simulink model "Battery_model_2D_Battery1"  (R2026a)
settings: Solver=VariableStepAuto  StopTime=10000
InitFcn:
  | %% Universal Parameters
  | 
  | Cycle_num = 1000; % number of cycles
  | 
  | Temp_state = 35;
  | 
  | 
  | SoC_state = 0.5;
  | 
  | OCV = [ 3.0025,3.4635,3.521,3.5618,3.6058,3.6426,3.6725,3.7049,3.7486,3.79951,3.8418,3.8738 ,3.9044,3.9448,3.9813,4.0222 ,4.0498,4.0658,4.0919,4.1359,4.2];
  | 
  | 
  | % Cn = 540; % As
  | Ru = 3.19; % KW^-1
  | Rc = 1.94; % KW^-1
  | Cc = 62.7; % JK^-1
  | Cs = 4.5;  % JK^-1
  | 
  | Ea = 31500;  % J * mol^-1
  | eta = 152.5; % unitless
  | Ic = 9000;   % [1/s] normalized current rate
  | Rg = 8.314;  % J / K / mol
  | z = 0.57;    % Ah power law exponent
  | 
  | 
  | 
  | %% Breakpoints
  | Temp = [5, 15, 25, 35, 45];
  | SoC  = [0, 0.05, 0.10, 0.15, 0.20, 0.25, 0.30, 0.35, 0.40, 0.45, 0.50, 0.55, 0.60, 0.65, 0.70, 0.75, 0.80, 0.85, 0.90, 0.95, 1.00];
  | 
  | %% ── CHARGING Parameters ──────────────────────────────────────────────────────
  | 
  | % --- R0 (charge) ---
  | R0_5_ch  = [0.09098063, 0.09098063, 0.09098063, 0.07729039, 0.07041201, 0.07506999, 0.09974696 ...
  |              0.10355653, 0.10333513, 0.10371531, 0.10352259, 0.10328822, 0.10331602, 0.10342002 ...
  |              0.10364672, 0.10394453, 0.10423533, 0.10413898, 0.10372082, 0.10352712, 0.10300533];
  | R0_15_ch  = [0.12804680, 0.12804680, 0.12804680, 0.10877905, 0.09909838, 0.10565405, 0.14038460 ...
  |              0.14574622, 0.14543462, 0.14596969, 0.14569844, 0.14536859, 0.14540772, 0.14555409 ...
  |              0.14587315, 0.14629229, 0.14670156, 0.14656596, 0.14597744, 0.14570482, 0.14497046];
  | R0_25_ch  = [0.15714834, 0.15714834, 0.15714834, 0.13350157, 0.12162074, 0.12966634, 0.17229020 ...
  |              0.17887036, 0.17848795, 0.17914462, 0.17881173, 0.17840691, 0.17845493, 0.17863457 ...
  |              0.17902614, 0.17954054, 0.18004283, 0.17987641, 0.17915414, 0.17881956, 0.17791829];
  | R0_35_ch  = [0.19207020, 0.19207020, 0.19207020, 0.16316858, 0.14864757, 0.15848107, 0.21057691 ...
  |              0.21861932, 0.21815193, 0.21895454, 0.21854766, 0.21805289, 0.21811158, 0.21833114 ...
  |              0.21880973, 0.21943844, 0.22005234, 0.21984894, 0.21896616, 0.21855723, 0.21745569];
  | R0_45_ch  = [0.21607897, 0.21607897, 0.21607897, 0.18356466, 0.16722852, 0.17829121, 0.23689902 ...
  |              0.24594674, 0.24542093, 0.24632386, 0.24586613, 0.24530950, 0.24537554, 0.24562254 ...
  |              0.24616095, 0.24686825, 0.24755889, 0.24733007, 0.24633694, 0.24587689, 0.24463765];
  | R0_ch = [R0_5_ch; R0_15_ch; R0_25_ch; R0_35_ch; R0_45_ch];
  | 
  | % --- R1 (charge) ---
  | R1_5_ch  = [0.02042370, 0.02042370, 0.02077370, 0.01704263, 0.01499740, 0.01607981, 0.02204645 ...
  |              0.02311272, 0.02295408, 0.02251460, 0.02241361, 0.02224373, 0.02204869, 0.02198763 ...
  |              0.02193720, 0.02188186, 0.02186556, 0.02196136, 0.02204788, 0.02216615, 0.02233881];
  | R1_15_ch  = [0.03713400, 0.03713400, 0.03777036, 0.03098661, 0.02726801, 0.02923601, 0.04008445 ...
  |              0.04202312, 0.04173470, 0.04093563, 0.04075202, 0.04044315, 0.04008853, 0.03997751 ...
  |              0.03988582, 0.03978519, 0.03975555, 0.03992974, 0.04008704, 0.04030208, 0.04061602];
  | R1_25_ch  = [0.05835343, 0.05835343, 0.05935343, 0.04869324, 0.04284973, 0.04594231, 0.06298985 ...
  |              0.06603633, 0.06558310, 0.06432742, 0.06403890, 0.06355352, 0.06299626, 0.06282180 ...
  |              0.06267773, 0.06251959, 0.06247302, 0.06274674, 0.06299393, 0.06333184, 0.06382517];
  | R1_35_ch  = [0.08169480, 0.08169480, 0.08309480, 0.06817054, 0.05998962, 0.06431924, 0.08818579 ...
  |              0.09245087, 0.09181634, 0.09005839, 0.08965446, 0.08897493, 0.08819477, 0.08795052 ...
  |              0.08774882, 0.08752743, 0.08746222, 0.08784544, 0.08819150, 0.08866458, 0.08935524];
  | R1_45_ch  = [0.09283500, 0.09283500, 0.09442590, 0.07746652, 0.06817002, 0.07309004, 0.10021113 ...
  |              0.10505781, 0.10433675, 0.10233908, 0.10188006, 0.10110787, 0.10022133, 0.09994378 ...
  |              0.09971457, 0.09946299, 0.09938889, 0.09982437, 0.10021762, 0.10075521, 0.10154005];
  | R1_ch = [R1_5_ch; R1_15_ch; R1_25_ch; R1_35_ch; R1_45_ch];
  | 
  | % --- C1 (charge) ---
  | C1_5_ch  = [0.00131968, 0.00131968, 0.00371968, 0.00485103, 0.00496080, 0.00442106, 0.00227620 ...
  |              0.00183668, 0.00180689, 0.00187453, 0.00180955, 0.00174851, 0.00174631, 0.00176395 ...
  |              0.00179412, 0.00181842, 0.00185225, 0.00188926, 0.00185128, 0.00180647, 0.00169075];
  | C1_15_ch  = [0.00079181, 0.00079181, 0.00223181, 0.00291062, 0.00297648, 0.00265264, 0.00136572 ...
  |              0.00110201, 0.00108413, 0.00112472, 0.00108573, 0.00104911, 0.00104778, 0.00105837 ...
  |              0.00107647, 0.00109105, 0.00111135, 0.00113356, 0.00111077, 0.00108388, 0.00101445];
  | C1_25_ch  = [0.00054987, 0.00054987, 0.00154987, 0.00202126, 0.00206700, 0.00184211, 0.00094842 ...
  |              0.00076528, 0.00075287, 0.00078105, 0.00075398, 0.00072855, 0.00072763, 0.00073498 ...
  |              0.00074755, 0.00075768, 0.00077177, 0.00078719, 0.00077137, 0.00075270, 0.00070448];
  | C1_35_ch  = [0.00040398, 0.00040398, 0.00113868, 0.00148501, 0.00151861, 0.00135339, 0.00069680 ...
  |              0.00056225, 0.00055313, 0.00057383, 0.00055394, 0.00053526, 0.00053458, 0.00053998 ...
  |              0.00054922, 0.00055666, 0.00056701, 0.00057834, 0.00056672, 0.00055300, 0.00051758];
  | C1_45_ch  = [0.00035348, 0.00035348, 0.00099634, 0.00129938, 0.00132879, 0.00118421, 0.00060970 ...
  |              0.00049197, 0.00048399, 0.00050210, 0.00048470, 0.00046835, 0.00046776, 0.00047249 ...
  |              0.00048057, 0.00048708, 0.00049614, 0.00050605, 0.00049588, 0.00048388, 0.00045288];
  | C1_ch = [C1_5_ch; C1_15_ch; C1_25_ch; C1_35_ch; C1_45_ch];
  | 
  | % --- R2 (charge) ---
  | R2_5_ch  = [0.11513467, 0.11513467, 0.11572467, 0.08930958, 0.07499462, 0.08137577, 0.11786696 ...
  |              0.12356614, 0.12135259, 0.11255792, 0.11155202, 0.10963847, 0.10666546, 0.10530908 ...
  |              0.10344252, 0.10111039, 0.09966464, 0.09882254, 0.09857888, 0.09907923, 0.10050567];
  | R2_15_ch  = [0.15351291, 0.15351291, 0.15429957, 0.11907944, 0.09999283, 0.10850103, 0.15715596 ...
  |              0.16475486, 0.16180346, 0.15007724, 0.14873603, 0.14618463, 0.14222061, 0.14041211 ...
  |              0.13792336, 0.13481386, 0.13288620, 0.13176339, 0.13143851, 0.13210565, 0.13400756];
  | R2_25_ch  = [0.19514352, 0.19514352, 0.19614352, 0.15137217, 0.12710953, 0.13792503, 0.19977451 ...
  |              0.20943414, 0.20568235, 0.19077614, 0.18907121, 0.18582791, 0.18078891, 0.17848997 ...
  |              0.17532630, 0.17137355, 0.16892312, 0.16749583, 0.16708284, 0.16793090, 0.17034859];
  | R2_35_ch  = [0.23026935, 0.23026935, 0.23144935, 0.17861916, 0.14998924, 0.16275153, 0.23573393 ...
  |              0.24713228, 0.24270518, 0.22511585, 0.22310403, 0.21927693, 0.21333091, 0.21061816 ...
  |              0.20688503, 0.20222079, 0.19932929, 0.19764508, 0.19715775, 0.19815847, 0.20101134];
  | R2_45_ch  = [0.23026935, 0.23026935, 0.23144935, 0.17861916, 0.14998924, 0.16275153, 0.23573393 ...
  |              0.24713228, 0.24270518, 0.22511585, 0.22310403, 0.21927693, 0.21333091, 0.21061816 ...
  |              0.20688503, 0.20222079, 0.19932929, 0.19764508, 0.19715775, 0.19815847, 0.20101134];
  | R2_ch = [R2_5_ch; R2_15_ch; R2_25_ch; R2_35_ch; R2_45_ch];
  | 
  | % --- C2 (charge) ---
  | C2_5_ch  = [0.03008769, 0.03008769, 0.03168769, 0.03903172, 0.04044082, 0.03636374, 0.02171253 ...
  |              0.01875550, 0.01849351, 0.01861683, 0.01820564, 0.01769637, 0.01745594, 0.01745402 ...
  |              0.01764677, 0.01786246, 0.01804175, 0.01818826, 0.01806588, 0.01791416, 0.01753917];
  | C2_15_ch  = [0.02507307, 0.02507307, 0.02640641, 0.03252643, 0.03370068, 0.03030312, 0.01809378 ...
  |              0.01562958, 0.01541126, 0.01551402, 0.01517136, 0.01474698, 0.01454661, 0.01454501 ...
  |              0.01470564, 0.01488538, 0.01503480, 0.01515688, 0.01505490, 0.01492846, 0.01461597];
  | C2_25_ch  = [0.01880481, 0.01880481, 0.01980481, 0.02439482, 0.02527551, 0.02272734, 0.01357033 ...
  |              0.01172219, 0.01155844, 0.01163552, 0.01137852, 0.01106023, 0.01090996, 0.01090876 ...
  |              0.01102923, 0.01116404, 0.01127610, 0.01136766, 0.01129117, 0.01119635, 0.01096198];
  | C2_35_ch  = [0.01002923, 0.01002923, 0.01056256, 0.01301057, 0.01348027, 0.01212125, 0.00723751 ...
  |              0.00625183, 0.00616450, 0.00620561, 0.00606854, 0.00589879, 0.00581865, 0.00581800 ...
  |              0.00588225, 0.00595415, 0.00601392, 0.00606275, 0.00602196, 0.00597138, 0.00584639];
  | C2_45_ch  = [0.00578609, 0.00578609, 0.00609379, 0.00750610, 0.00777708, 0.00699303, 0.00417549 ...
  |              0.00360683, 0.00355644, 0.00358016, 0.00350108, 0.00340315, 0.00335691, 0.00335654 ...
  |              0.00339361, 0.00343509, 0.00346957, 0.00349774, 0.00347421, 0.00344503, 0.00337292];
  | C2_ch = [C2_5_ch; C2_15_ch; C2_25_ch; C2_35_ch; C2_45_ch];
  | 
  | %% ── DISCHARGING Parameters ──────────────────────────────────────────────────
  | 
  | % --- R0 (discharge) ---
  | R0_5_dis = [0.10989020, 0.10989020, 0.10613356, 0.10505533, 0.10472760, 0.10437825, 0.10404639 ...
  |              0.10374473, 0.10354188, 0.10380928, 0.10392383, 0.10370969, 0.10380887, 0.10406384 ...
  |              0.10362800, 0.10289786, 0.10271463, 0.10291492, 0.10291492, 0.10291492, 0.10291492];
  | R0_15_dis = [0.15466028, 0.15466028, 0.14937315, 0.14785565, 0.14739440, 0.14690272, 0.14643566 ...
  |              0.14601111, 0.14572561, 0.14610195, 0.14626317, 0.14596178, 0.14610137, 0.14646022 ...
  |              0.14584681, 0.14481920, 0.14456133, 0.14484322, 0.14484322, 0.14484322, 0.14484322];
  | R0_25_dis = [0.18981035, 0.18981035, 0.18332160, 0.18145921, 0.18089313, 0.18028970, 0.17971650 ...
  |              0.17919545, 0.17884507, 0.17930694, 0.17950479, 0.17913491, 0.17930622, 0.17974663 ...
  |              0.17899382, 0.17773266, 0.17741618, 0.17776213, 0.17776213, 0.17776213, 0.17776213];
  | R0_35_dis = [0.23199043, 0.23199043, 0.22405973, 0.22178348, 0.22109160, 0.22035408, 0.21965349 ...
  |              0.21901666, 0.21858841, 0.21915293, 0.21939475, 0.21894267, 0.21915205, 0.21969033 ...
  |              0.21877022, 0.21722881, 0.21684200, 0.21726483, 0.21726483, 0.21726483, 0.21726483];
  | R0_45_dis = [0.26098923, 0.26098923, 0.25206720, 0.24950641, 0.24872805, 0.24789834, 0.24711018 ...
  |              0.24639374, 0.24591197, 0.24654705, 0.24681909, 0.24631051, 0.24654606, 0.24715162 ...
  |              0.24611650, 0.24438241, 0.24394725, 0.24442293, 0.24442293, 0.24442293, 0.24442293];
  | R0_dis = [R0_5_dis; R0_15_dis; R0_25_dis; R0_35_dis; R0_45_dis];
  | 
  | % --- R1 (discharge) ---
  | R1_5_dis = [0.02375913, 0.02375913, 0.02346547, 0.02303791, 0.02231945, 0.02189989, 0.02144243 ...
  |              0.02130311, 0.02160261, 0.02181022, 0.02148990, 0.02114871, 0.02118288, 0.02122248 ...
  |              0.02108587, 0.02096272, 0.02103812, 0.02147206, 0.02147206, 0.02147206, 0.02147206];
  | R1_15_dis = [0.04319842, 0.04319842, 0.04266449, 0.04188712, 0.04058082, 0.03981799, 0.03898623 ...
  |              0.03873294, 0.03927746, 0.03965494, 0.03907254, 0.03845219, 0.03851432, 0.03858632 ...
  |              0.03833794, 0.03811403, 0.03825113, 0.03904011, 0.03904011, 0.03904011, 0.03904011];
  | R1_25_dis = [0.06788323, 0.06788323, 0.06704419, 0.06582261, 0.06376986, 0.06257113, 0.06126407 ...
  |              0.06086604, 0.06172173, 0.06231490, 0.06139971, 0.06042488, 0.06052251, 0.06063565 ...
  |              0.06024533, 0.05989348, 0.06010892, 0.06134875, 0.06134875, 0.06134875, 0.06134875];
  | R1_35_dis = [0.09503652, 0.09503652, 0.09386187, 0.09215166, 0.08927780, 0.08759958, 0.08576970 ...
  |              0.08521246, 0.08641042, 0.08724086, 0.08595959, 0.08459483, 0.08473151, 0.08488991 ...
  |              0.08434347, 0.08385087, 0.08415248, 0.08588825, 0.08588825, 0.08588825, 0.08588825];
  | R1_45_dis = [0.10799604, 0.10799604, 0.10666122, 0.10471780, 0.10145205, 0.09954498, 0.09746557 ...
  |              0.09683234, 0.09819366, 0.09913734, 0.09768135, 0.09613048, 0.09628581, 0.09646581 ...
  |              0.09584485, 0.09528508, 0.09562782, 0.09760029, 0.09760029, 0.09760029, 0.09760029];
  | R1_dis = [R1_5_dis; R1_15_dis; R1_25_dis; R1_35_dis; R1_45_dis];
  | 
  | % --- C1 (discharge) ---
  | C1_5_dis = [0.00252928, 0.00252928, 0.00249315, 0.00245948, 0.00240651, 0.00234416, 0.00222824 ...
  |              0.00216919, 0.00209708, 0.00206633, 0.00204028, 0.00201931, 0.00208776, 0.00216878 ...
  |              0.00213557, 0.00205949, 0.00202298, 0.00197302, 0.00197302, 0.00197302, 0.00197302];
  | C1_15_dis = [0.00151757, 0.00151757, 0.00149589, 0.00147569, 0.00144390, 0.00140650, 0.00133695 ...
  |              0.00130151, 0.00125825, 0.00123980, 0.00122417, 0.00121159, 0.00125266, 0.00130127 ...
  |              0.00128134, 0.00123569, 0.00121379, 0.00118381, 0.00118381, 0.00118381, 0.00118381];
  | C1_25_dis = [0.00105387, 0.00105387, 0.00103881, 0.00102478, 0.00100271, 0.00097673, 0.00092843 ...
  |              0.00090383, 0.00087378, 0.00086097, 0.00085012, 0.00084138, 0.00086990, 0.00090366 ...
  |              0.00088982, 0.00085812, 0.00084291, 0.00082209, 0.00082209, 0.00082209, 0.00082209];
  | C1_35_dis = [0.00077427, 0.00077427, 0.00076321, 0.00075290, 0.00073669, 0.00071760, 0.00068212 ...
  |              0.00066404, 0.00064196, 0.00063255, 0.00062457, 0.00061816, 0.00063911, 0.00066391 ...
  |              0.00065375, 0.00063046, 0.00061928, 0.00060398, 0.00060398, 0.00060398, 0.00060398];
  | C1_45_dis = [0.00067749, 0.00067749, 0.00066781, 0.00065879, 0.00064460, 0.00062790, 0.00059685 ...
  |              0.00058103, 0.00056172, 0.00055348, 0.00054650, 0.00054089, 0.00055922, 0.00058092 ...
  |              0.00057203, 0.00055165, 0.00054187, 0.00052849, 0.00052849, 0.00052849, 0.00052849];
  | C1_dis = [C1_5_dis; C1_15_dis; C1_25_dis; C1_35_dis; C1_45_dis];
  | 
  | % --- R2 (discharge) ---
  | R2_5_dis = [0.12377240, 0.12377240, 0.12499052, 0.12084607, 0.11292650, 0.10875026, 0.10601660 ...
  |              0.10536563, 0.10667297, 0.10779017, 0.10371058, 0.09898872, 0.09840504, 0.09800231 ...
  |              0.09623862, 0.09363203, 0.09353319, 0.09588010, 0.09588010, 0.09588010, 0.09588010];
  | R2_15_dis = [0.16502986, 0.16502986, 0.16665402, 0.16112809, 0.15056867, 0.14500034, 0.14135547 ...
  |              0.14048751, 0.14223062, 0.14372022, 0.13828077, 0.13198496, 0.13120672, 0.13066974 ...
  |              0.12831816, 0.12484271, 0.12471092, 0.12784013, 0.12784013, 0.12784013, 0.12784013];
  | R2_25_dis = [0.20978372, 0.20978372, 0.21184834, 0.20482384, 0.19140085, 0.18432247, 0.17968916 ...
  |              0.17858582, 0.18080164, 0.18269520, 0.17578065, 0.16777749, 0.16678821, 0.16610560 ...
  |              0.16311630, 0.15869836, 0.15853083, 0.16250864, 0.16250864, 0.16250864, 0.16250864];
  | R2_35_dis = [0.24754479, 0.24754479, 0.24998104, 0.24169213, 0.22585300, 0.21750051, 0.21203321 ...
  |              0.21073127, 0.21334594, 0.21558033, 0.20742116, 0.19797744, 0.19681009, 0.19600461 ...
  |              0.19247724, 0.18726407, 0.18706638, 0.19176020, 0.19176020, 0.19176020, 0.19176020];
  | R2_45_dis = [0.24754479, 0.24754479, 0.24998104, 0.24169213, 0.22585300, 0.21750051, 0.21203321 ...
  |              0.21073127, 0.21334594, 0.21558033, 0.20742116, 0.19797744, 0.19681009, 0.19600461 ...
  |              0.19247724, 0.18726407, 0.18706638, 0.19176020, 0.19176020, 0.19176020, 0.19176020];
  | R2_dis = [R2_5_dis; R2_15_dis; R2_25_dis; R2_35_dis; R2_45_dis];
  | 
  | % --- C2 (discharge) ---
  | C2_5_dis = [0.02652842, 0.02652842, 0.02631500, 0.02521431, 0.02331166, 0.02179726, 0.02020022 ...
  |              0.01939438, 0.01937170, 0.01943623, 0.01914013, 0.01889522, 0.01909655, 0.01931546 ...
  |              0.01917944, 0.01895760, 0.01881918, 0.01863074, 0.01863074, 0.01863074, 0.01863074];
  | C2_15_dis = [0.02210702, 0.02210702, 0.02192916, 0.02101192, 0.01942638, 0.01816439, 0.01683351 ...
  |              0.01616198, 0.01614308, 0.01619686, 0.01595011, 0.01574602, 0.01591379, 0.01609622 ...
  |              0.01598286, 0.01579800, 0.01568265, 0.01552562, 0.01552562, 0.01552562, 0.01552562];
  | C2_25_dis = [0.01658027, 0.01658027, 0.01644687, 0.01575894, 0.01456979, 0.01362329, 0.01262514 ...
  |              0.01212149, 0.01210731, 0.01214764, 0.01196258, 0.01180951, 0.01193535, 0.01207217 ...
  |              0.01198715, 0.01184850, 0.01176199, 0.01164421, 0.01164421, 0.01164421, 0.01164421];
  | C2_35_dis = [0.00884281, 0.00884281, 0.00877167, 0.00840477, 0.00777055, 0.00726575, 0.00673341 ...
  |              0.00646479, 0.00645723, 0.00647874, 0.00638004, 0.00629841, 0.00636552, 0.00643849 ...
  |              0.00639315, 0.00631920, 0.00627306, 0.00621025, 0.00621025, 0.00621025, 0.00621025];
  | C2_45_dis = [0.00510162, 0.00510162, 0.00506058, 0.00484890, 0.00448301, 0.00419178, 0.00388466 ...
  |              0.00372969, 0.00372533, 0.00373774, 0.00368079, 0.00363370, 0.00367241, 0.00371451 ...
  |              0.00368835, 0.00364569, 0.00361907, 0.00358283, 0.00358283, 0.00358283, 0.00358283];
  | C2_dis = [C2_5_dis; C2_15_dis; C2_25_dis; C2_35_dis; C2_45_dis];
model workspace (MAT data in the model file):
  C_As = 150
  Cn = 150
  I_c = 1
  I_c_full_charged = 0.0333333333333
  Tc_state = 35.0044118318
  Ts_state = 35.0027406087
  V1_state = 0.00398713164124
  V2_state = 0.00927212980774
  V_cutoff = 3
  V_max = 4.2
  current_SoC = 0.996576803874
undefined symbols (not defined in the file): V1_ini
libraries: simulink x7
(part 1 of 2)
settings Model: Creator=vatan  LastModifiedBy=beaga
settings DebuggingCC: UnderspecifiedInitializationDetection=Classic
settings SimscapeCC: SimscapeNominalValues="[{\"value\":\"1\",\"unit\":\"A\"},{\"value\":\"1\",\"unit\":\"bar\"},{\"value\":\"1\",\"unit\":\"cm^2\"},{\"value\":\"1\",\"unit\":\"cm^3/s\"},{\"value\":\"1\",\"unit\":\"kJ/kg\"},{\"value\":\"1\",\"unit\":\"kW\"},{\"value\":\"1\",\"unit\":\"l\"},{\"value\":\"1\",\"unit\":\"N\"},{\"value\":\"1\",\"unit\":\"N*m\"},{\"value\":\"1\",\"unit\":\"V\"}]"  SimscapeLogType=none  SimscapeLogDataHistory=5000.0

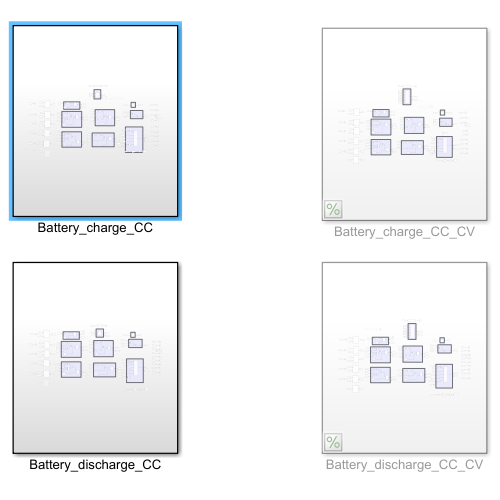
[thumbnail: Simulink's stored preview of the top-level diagram]
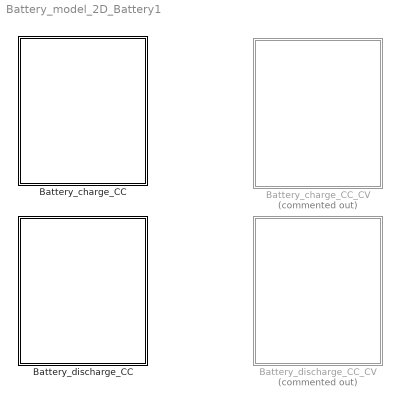
== system Battery_model_2D_Battery1 ==
  Battery_charge_CC : Subsystem
  Battery_charge_CC_CV : Subsystem  Commented=on
  Battery_discharge_CC : Subsystem
  Battery_discharge_CC_CV : Subsystem  Commented=on

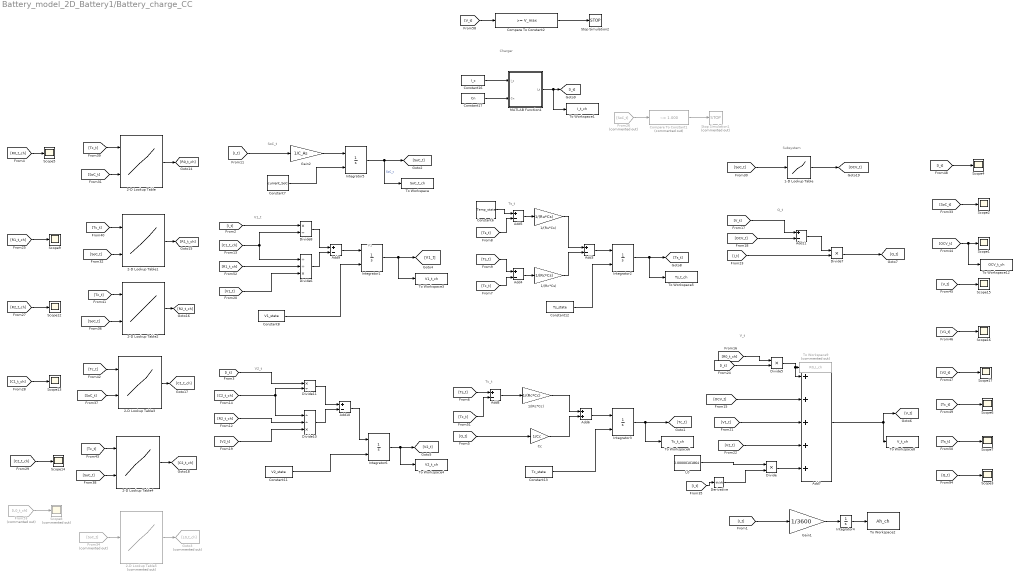
== system Battery_model_2D_Battery1/Battery_charge_CC ==
  note: Subsystem
  note: Tc_t
  note: Ts_t
  note: V_t
  note: V2_t
  note: V1_t
  note: SoC_t
  note: V1
  note: Q_t
  note: Charger
  1-D Lookup Table : Lookup_n-D  NumberOfTableDimensions=1  BreakpointsForDimension1=SoC  BreakpointsForDimension2=Temp  Table=OCV  InternalRulePriority=Speed  RndMeth=Simplest
  1/(Rc*Cc) : Gain  Gain=1/(Rc*Cc)
  1/(Rc*Cs) : Gain  Gain=1/(Rc*Cs)
  1/(Ru*Cs) : Gain  Gain=1/(Ru*Cs)
  2-D Lookup Table : Lookup_n-D  BreakpointsForDimension1=Temp  BreakpointsForDimension2=SoC  Table=R0_ch  InternalRulePriority=Speed  RndMeth=Simplest
      settings: InputPortMap=u0,u1
  2-D Lookup Table1 : Lookup_n-D  BreakpointsForDimension1=Temp  BreakpointsForDimension2=SoC  Table=R1_ch  InternalRulePriority=Speed  RndMeth=Simplest
      settings: InputPortMap=u0,u1
  2-D Lookup Table2 : Lookup_n-D  BreakpointsForDimension1=Temp  BreakpointsForDimension2=SoC  Table=R2_ch  InternalRulePriority=Speed  RndMeth=Simplest
      settings: InputPortMap=u0,u1
  2-D Lookup Table3 : Lookup_n-D  BreakpointsForDimension1=Temp  BreakpointsForDimension2=SoC  Table=C1_ch  InternalRulePriority=Speed  RndMeth=Simplest
      settings: InputPortMap=u0,u1
  2-D Lookup Table4 : Lookup_n-D  BreakpointsForDimension1=Temp  BreakpointsForDimension2=SoC  Table=C2_ch  InternalRulePriority=Speed  RndMeth=Simplest
      settings: InputPortMap=u0,u1
  2-D Lookup Table5 : Lookup_n-D  Commented=on  NumberOfTableDimensions=1  BreakpointsForDimension1=Temp  BreakpointsForDimension2=SoC  Table=C2_ch  InternalRulePriority=Speed  RndMeth=Simplest
  Add{3..5,8..11} (7 alike) : Sum  Inputs=+-
  Add6 : Sum
  Add7 : Sum  Inputs=+++++
  Cc : Gain  Gain=1/Cc
  Compare To Constant1 : simulink/Logic and Bit Operations/Compare To Constant  Commented=on  relop=~=  const=1.000  OutDataTypeStr=boolean
  Compare To Constant2 : simulink/Logic and Bit Operations/Compare To Constant  relop=>=  const=V_max  OutDataTypeStr=boolean
  Constant11 : Constant  Value=V2_state
  Constant12 : Constant  Value=Ts_state
  Constant13 : Constant  Value=Tc_state
  Constant16 : Constant  Value=I_c
  Constant17 : Constant  Value=Cn
  Constant6 : Constant  Value=Temp_state
  Constant7 : Constant  Value=current_SoC
  Constant8 : Constant  Value=V1_state
  Derivative : Derivative
  Divide : Product  Inputs=**
  Divide10 : Product  Inputs=//*
  Divide11 : Product  Inputs=*/
  Divide5 : Product  Inputs=**
  Divide6 : Product  Inputs=//*
  Divide7 : Product  Inputs=**
  Divide8 : Product  Inputs=*/
  From26 : From  Commented=on  GotoTag=SoC_t
  From34 : From  Commented=on  GotoTag=SoC_t
  From53 : From  Commented=on  GotoTag=L0_t_ch
  Gain1 : Gain  Gain=1/3600
  Gain2 : Gain  Gain=1/C_As
  Goto3 : Goto  Commented=on  GotoTag=L0_t_ch
  Integrator{1..3,6} (4 alike) : Integrator  InitialConditionSource=external
  Integrator4 : Integrator
  Integrator5 : Integrator  InitialConditionSource=external  InitialCondition=V1_ini
  L0 : Constant  Value=0.00000101864
  MATLAB Function4 : MATLAB Function  TreatAsAtomicUnit=on
  Scope{1..7,9,12..17} (14 alike) : Scope
      Scope1 settings: ActiveDisplayYMinimum=2.2604  ActiveDisplayYMaximum=3.6664  DataLoggingVariableName=ScopeData7
      Scope12 settings: ActiveDisplayYMinimum=0.00751  ActiveDisplayYMaximum=0.04204  DataLoggingVariableName=ScopeData3
      Scope13 settings: ActiveDisplayYMinimum=1446.0874  ActiveDisplayYMaximum=2982.5444  DataLoggingVariableName=ScopeData4
      Scope14 settings: ActiveDisplayYMinimum=14445.3812  ActiveDisplayYMaximum=112360.8817  DataLoggingVariableName=ScopeData5
      Scope15 settings: ActiveDisplayYMinimum=2.15  ActiveDisplayYMaximum=4.15  DataLoggingVariableName=ScopeData8
      Scope16 settings: ActiveDisplayYMinimum=-0.00306  ActiveDisplayYMaximum=0.0275  DataLoggingVariableName=ScopeData9
      Scope17 settings: ActiveDisplayYMinimum=-0.00274  ActiveDisplayYMaximum=0.02463  DataLoggingVariableName=ScopeData10
      Scope2 settings: ActiveDisplayYMinimum=0.0058466  ActiveDisplayYMaximum=0.025847  DataLoggingVariableName=ScopeData6
      Scope3 settings: ActiveDisplayYMinimum=-7.8351  ActiveDisplayYMaximum=6.6118  DataLoggingVariableName=ScopeData14
      Scope4 settings: ActiveDisplayYMinimum=0.049838  ActiveDisplayYMaximum=0.24984  DataLoggingVariableName=ScopeData11
      Scope5 settings: ActiveDisplayYMinimum=0.00753  ActiveDisplayYMaximum=0.01894
      Scope6 settings: ActiveDisplayYMinimum=24.9953  ActiveDisplayYMaximum=44.9953  DataLoggingVariableName=ScopeData12
      Scope7 settings: ActiveDisplayYMinimum=-5.0616  ActiveDisplayYMaximum=45.5546  DataLoggingVariableName=ScopeData13
      Scope9 settings: ActiveDisplayYMinimum=0.00821  ActiveDisplayYMaximum=0.03092  DataLoggingVariableName=ScopeData2
  Scope8 : Scope  Commented=on
      settings: ActiveDisplayYMinimum=14445.3812  ActiveDisplayYMaximum=112360.8817  DataLoggingVariableName=ScopeData24
  Stop Simulation1 : Stop  Commented=on
  Stop Simulation2 : Stop
  To Workspace : ToWorkspace  VariableName=SoC_t_ch  SampleTime=-1
      settings: Save2DSignal=2-D array (concatenate along first dimension)
  To Workspace1 : ToWorkspace  VariableName=I_t_ch  SaveFormat=Timeseries  SampleTime=-1
      settings: Save2DSignal=2-D array (concatenate along first dimension)
  To Workspace12 : ToWorkspace  VariableName=OCV_t_ch  SampleTime=-1
      settings: Save2DSignal=2-D array (concatenate along first dimension)
  To Workspace2 : ToWorkspace  VariableName=Ah_ch  SampleTime=-1
      settings: Save2DSignal=2-D array (concatenate along first dimension)
  To Workspace3 : ToWorkspace  VariableName=V1_t_ch  SampleTime=-1
      settings: Save2DSignal=2-D array (concatenate along first dimension)
  To Workspace4 : ToWorkspace  VariableName=V2_t_ch  SampleTime=-1
      settings: Save2DSignal=2-D array (concatenate along first dimension)
  To Workspace5 : ToWorkspace  VariableName=Ts_t_ch  SampleTime=-1
      settings: Save2DSignal=2-D array (concatenate along first dimension)
  To Workspace6 : ToWorkspace  VariableName=Tc_t_ch  SampleTime=-1
      settings: Save2DSignal=2-D array (concatenate along first dimension)
  To Workspace8 : ToWorkspace  VariableName=V_t_ch  SaveFormat=Timeseries  SampleTime=-1
      settings: Save2DSignal=2-D array (concatenate along first dimension)
  To Workspace9 : ToWorkspace  Commented=on  VariableName=R0_I_ch  SampleTime=-1
      settings: Save2DSignal=2-D array (concatenate along first dimension)
  wires:
  Divide10/1 -> Add10/2
  Add5/1 -> 1/(Ru*Cs)/1
  Add11/1 -> Divide7/1
  [Tc_t] -> Add4/2
  1/(Rc*Cc)/1 -> Add6/1
  [V2_t] -> Add7/4
  Divide5/1 -> Add7/1, To Workspace9/1
  Add4/1 -> 1/(Rc*Cs)/1
  Divide6/1 -> Add9/2
  [I_t] -> Divide11/1
  [Tc_t] -> 2-D Lookup Table2/1
  Cc/1 -> Add6/2
  [Tc_t] -> 2-D Lookup Table/1
  Divide7/1 -> [Q_t]
  1-D Lookup Table/1 -> [OCV_t]
  [SoC_t] -> 2-D Lookup Table1/2
  2-D Lookup Table3/1 -> [C1_t_ch]
  [V2_t] -> Scope17/1
  Add9/1 -> Integrator1/1
  2-D Lookup Table/1 -> [R0_t_ch]
  [Ts_t] -> Scope7/1
  [I_t] -> Scope4/1
  [V2_t] -> Divide10/3
  [R1_t_ch] -> Scope9/1
  Add10/1 -> Integrator6/1
  2-D Lookup Table4/1 -> [C2_t_ch]
  [SoC_t] -> 1-D Lookup Table/1
  [R0_t_ch] -> Scope5/1
  [SoC_t] -> 2-D Lookup Table/2
  [R0_t_ch] -> Divide5/1
  [I_t] -> Divide7/2
  [V1_t] -> Scope16/1
  [C2_t_ch] -> Divide10/1, Divide11/2
  Add3/1 -> Integrator2/1
  [V_t] -> Add11/1
  [Q_t] -> Scope3/1
  [I_t] -> Divide5/2
  [SoC_t] -> 2-D Lookup Table3/2
  1/(Rc*Cs)/1 -> Add3/2
  [OCV_t] -> To Workspace12/1, Scope1/1
  [C1_t_ch] -> Scope13/1
  [Tc_t] -> Scope6/1
  Divide8/1 -> Add9/1
  [OCV_t] -> Add11/2
  [V1_t] -> Divide6/3
  [Ts_t] -> Add4/1
  [Tc_t] -> 2-D Lookup Table1/1
  [C1_t_ch] -> Divide8/2, Divide6/1
  [Tc_t] -> 2-D Lookup Table3/1
  Gain2/1 -> Integrator5/1
  Add8/1 -> 1/(Rc*Cc)/1
  [R1_t_ch] -> Divide6/2
  [R2_t_ch] -> Scope12/1
  [Q_t] -> Cc/1
  Add6/1 -> Integrator3/1
  [R2_t_ch] -> Divide10/2
  [Ts_t] -> Add8/1
  2-D Lookup Table2/1 -> [R2_t_ch]
  Divide11/1 -> Add10/1
  [C2_t_ch] -> Scope14/1
  Add7/1 -> To Workspace8/1, [V_t]
  [SoC_t] -> 2-D Lookup Table2/2
  Integrator3/1 -> To Workspace6/1, [Tc_t]
  [Ts_t] -> Add5/2
  [Tc_t] -> Add8/2
  [I_t] -> Divide8/1
  Integrator6/1 -> To Workspace4/1, [V2_t]
  Integrator5/1 -> To Workspace/1, [SoC_t]  "SoC_t"
  Integrator1/1 -> To Workspace3/1, [V1_t]
  [SoC_t] -> Scope2/1
  Constant6/1 -> Add5/1
  2-D Lookup Table1/1 -> [R1_t_ch]
  [V_t] -> Scope15/1
  [SoC_t] -> 2-D Lookup Table4/2
  1/(Ru*Cs)/1 -> Add3/1
  [I_t] -> Gain2/1
  [Tc_t] -> 2-D Lookup Table4/1
  [OCV_t] -> Add7/2
  [V1_t] -> Add7/3
  [I_t] -> Gain1/1
  Integrator4/1 -> To Workspace2/1
  Gain1/1 -> Integrator4/1
  Integrator2/1 -> To Workspace5/1, [Ts_t]
  From26/1 -> Compare To Constant1/1
  Compare To Constant1/1 -> Stop Simulation1/1
  Constant12/1 -> Integrator2/2
  Constant8/1 -> Integrator1/2
  Constant11/1 -> Integrator6/2
  Constant13/1 -> Integrator3/2
  Constant16/1 -> MATLAB Function4/1(I_c)
  Constant17/1 -> MATLAB Function4/2(Cn)
  [V_t] -> Compare To Constant2/1
  Compare To Constant2/1 -> Stop Simulation2/1
  MATLAB Function4/1(I_t) -> To Workspace1/1, [I_t]
  Constant7/1 -> Integrator5/2
  From34/1 -> 2-D Lookup Table5/1
  2-D Lookup Table5/1 -> Goto3/1
  From53/1 -> Scope8/1
  [I_t] -> Derivative/1
  L0/1 -> Divide/1
  Derivative/1 -> Divide/2
  Divide/1 -> Add7/5

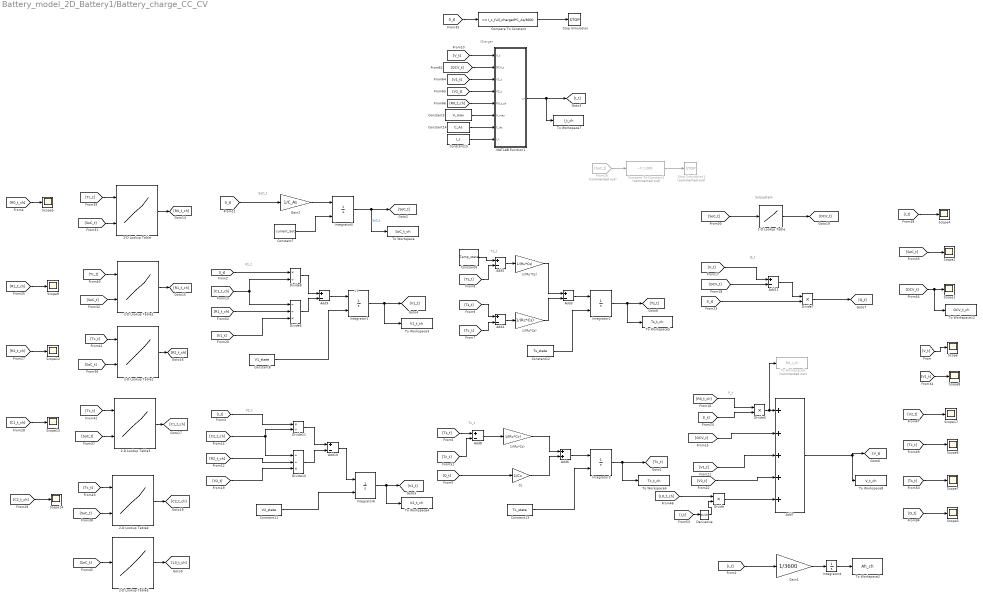
== system Battery_model_2D_Battery1/Battery_charge_CC_CV ==
  note: Subsystem
  note: Tc_t
  note: Ts_t
  note: V_t
  note: V2_t
  note: V1_t
  note: SoC_t
  note: V1
  note: Q_t
  note: Charger
  1-D Lookup Table : Lookup_n-D  NumberOfTableDimensions=1  BreakpointsForDimension1=SoC  BreakpointsForDimension2=Temp  Table=OCV  InternalRulePriority=Speed  RndMeth=Simplest
  1/(Rc*Cc) : Gain  Gain=1/(Rc*Cc)
  1/(Rc*Cs) : Gain  Gain=1/(Rc*Cs)
  1/(Ru*Cs) : Gain  Gain=1/(Ru*Cs)
  2-D Lookup Table : Lookup_n-D  BreakpointsForDimension1=Temp  BreakpointsForDimension2=SoC  Table=R0_ch  InternalRulePriority=Speed  RndMeth=Simplest
      settings: InputPortMap=u0,u1
  2-D Lookup Table1 : Lookup_n-D  BreakpointsForDimension1=Temp  BreakpointsForDimension2=SoC  Table=R1_ch  InternalRulePriority=Speed  RndMeth=Simplest
      settings: InputPortMap=u0,u1
  2-D Lookup Table2 : Lookup_n-D  BreakpointsForDimension1=Temp  BreakpointsForDimension2=SoC  Table=R2_ch  InternalRulePriority=Speed  RndMeth=Simplest
      settings: InputPortMap=u0,u1
  2-D Lookup Table3 : Lookup_n-D  BreakpointsForDimension1=Temp  BreakpointsForDimension2=SoC  Table=C1_ch  InternalRulePriority=Speed  RndMeth=Simplest
      settings: InputPortMap=u0,u1
  2-D Lookup Table4 : Lookup_n-D  BreakpointsForDimension1=Temp  BreakpointsForDimension2=SoC  Table=C2_ch  InternalRulePriority=Speed  RndMeth=Simplest
      settings: InputPortMap=u0,u1
  2-D Lookup Table5 : Lookup_n-D  NumberOfTableDimensions=1  BreakpointsForDimension1=Temp  BreakpointsForDimension2=SoC  Table=C2_ch  InternalRulePriority=Speed  RndMeth=Simplest
  Add{3..5,8..11} (7 alike) : Sum  Inputs=+-
  Add6 : Sum
  Add7 : Sum  Inputs=+++++
  Cc : Gain  Gain=1/Cc
  Compare To Constant : simulink/Logic and Bit Operations/Compare To Constant  relop=<=  const=I_c_full_charged*C_As/3600  OutDataTypeStr=boolean
  Compare To Constant1 : simulink/Logic and Bit Operations/Compare To Constant  Commented=on  relop=~=  const=1.000  OutDataTypeStr=boolean
  Constant11 : Constant  Value=V2_state
  Constant12 : Constant  Value=Ts_state
  Constant13 : Constant  Value=Tc_state
  Constant14 : Constant  Value=C_As
  Constant15 : Constant  Value=I_c
  Constant5 : Constant  Value=V_max
  Constant6 : Constant  Value=Temp_state
  Constant7 : Constant  Value=current_SoC
  Constant8 : Constant  Value=V1_state
  Derivative : Derivative
  Divide : Product  Inputs=**
  Divide10 : Product  Inputs=//*
  Divide11 : Product  Inputs=*/
  Divide5 : Product  Inputs=**
  Divide6 : Product  Inputs=//*
  Divide7 : Product  Inputs=**
  Divide8 : Product  Inputs=*/
  From26 : From  Commented=on  GotoTag=SoC_t
  Gain1 : Gain  Gain=1/3600
  Gain2 : Gain  Gain=1/C_As
  Integrator{1..3,6} (4 alike) : Integrator  InitialConditionSource=external
  Integrator4 : Integrator
  Integrator5 : Integrator  InitialConditionSource=external  InitialCondition=V1_ini
  MATLAB Function1 : MATLAB Function  TreatAsAtomicUnit=on
  Scope{,1..9,12..14,17} (14 alike) : Scope
      Scope settings: ActiveDisplayYMinimum=2.85883  ActiveDisplayYMaximum=4.3268
      Scope1 settings: ActiveDisplayYMinimum=2.85734  ActiveDisplayYMaximum=4.32322  DataLoggingVariableName=ScopeData7
      Scope12 settings: ActiveDisplayYMinimum=0.00751  ActiveDisplayYMaximum=0.04204  DataLoggingVariableName=ScopeData3
      Scope13 settings: ActiveDisplayYMinimum=1446.0874  ActiveDisplayYMaximum=2982.5444  DataLoggingVariableName=ScopeData4
      Scope14 settings: ActiveDisplayYMinimum=14445.3812  ActiveDisplayYMaximum=112360.8817  DataLoggingVariableName=ScopeData5
      Scope17 settings: ActiveDisplayYMinimum=-0.00038  ActiveDisplayYMaximum=0.00342  DataLoggingVariableName=ScopeData10
      Scope2 settings: ActiveDisplayYMinimum=0.00585  ActiveDisplayYMaximum=0.02585  DataLoggingVariableName=ScopeData6
      Scope3 settings: ActiveDisplayYMinimum=-0.00017  ActiveDisplayYMaximum=0.0017  DataLoggingVariableName=ScopeData14
      Scope4 settings: ActiveDisplayYMinimum=0.049838  ActiveDisplayYMaximum=0.24984  DataLoggingVariableName=ScopeData11
      Scope5 settings: ActiveDisplayYMinimum=0.00753  ActiveDisplayYMaximum=0.01894
      Scope6 settings: ActiveDisplayYMinimum=23.74914  ActiveDisplayYMaximum=36.2577  DataLoggingVariableName=ScopeData12
      Scope7 settings: ActiveDisplayYMinimum=23.74954  ActiveDisplayYMaximum=36.2541  DataLoggingVariableName=ScopeData13
      Scope8 settings: DataLoggingVariableName=ScopeData2
      Scope9 settings: ActiveDisplayYMinimum=0.00821  ActiveDisplayYMaximum=0.03092  DataLoggingVariableName=ScopeData2
  Stop Simulation : Stop
  Stop Simulation1 : Stop  Commented=on
  To Workspace : ToWorkspace  VariableName=SoC_t_ch  SampleTime=-1
      settings: Save2DSignal=2-D array (concatenate along first dimension)
  To Workspace12 : ToWorkspace  VariableName=OCV_t_ch  SampleTime=-1
      settings: Save2DSignal=2-D array (concatenate along first dimension)
  To Workspace2 : ToWorkspace  VariableName=Ah_ch  SampleTime=-1
      settings: Save2DSignal=2-D array (concatenate along first dimension)
  To Workspace3 : ToWorkspace  VariableName=V1_t_ch  SampleTime=-1
      settings: Save2DSignal=2-D array (concatenate along first dimension)
  To Workspace4 : ToWorkspace  VariableName=V2_t_ch  SampleTime=-1
      settings: Save2DSignal=2-D array (concatenate along first dimension)
  To Workspace5 : ToWorkspace  VariableName=Ts_t_ch  SampleTime=-1
      settings: Save2DSignal=2-D array (concatenate along first dimension)
  To Workspace6 : ToWorkspace  VariableName=Tc_t_ch  SampleTime=-1
      settings: Save2DSignal=2-D array (concatenate along first dimension)
  To Workspace7 : ToWorkspace  VariableName=I_t_ch  SaveFormat=Timeseries  SampleTime=-1
  To Workspace8 : ToWorkspace  VariableName=V_t_ch  SaveFormat=Timeseries  SampleTime=-1
      settings: Save2DSignal=2-D array (concatenate along first dimension)
  To Workspace9 : ToWorkspace  Commented=on  VariableName=R0_I_ch  SampleTime=-1
      settings: Save2DSignal=2-D array (concatenate along first dimension)
  wires:
  Divide10/1 -> Add10/2
  Add5/1 -> 1/(Ru*Cs)/1
  Add11/1 -> Divide7/1
  [Tc_t] -> Add4/2
  1/(Rc*Cc)/1 -> Add6/1
  [V2_t] -> Add7/4
  Divide5/1 -> To Workspace9/1, Add7/1
  Add4/1 -> 1/(Rc*Cs)/1
  Divide6/1 -> Add9/2
  [I_t] -> Divide11/1
  [Tc_t] -> 2-D Lookup Table2/1
  Cc/1 -> Add6/2
  [Tc_t] -> 2-D Lookup Table/1
  Divide7/1 -> [Q_t]
  1-D Lookup Table/1 -> [OCV_t]
  [SoC_t] -> 2-D Lookup Table1/2
  2-D Lookup Table3/1 -> [C1_t_ch]
  [V2_t] -> Scope17/1
  Add9/1 -> Integrator1/1
  2-D Lookup Table/1 -> [R0_t_ch]
  [Ts_t] -> Scope7/1
  [I_t] -> Scope4/1
  [V2_t] -> Divide10/3
  [R1_t_ch] -> Scope9/1
  Add10/1 -> Integrator6/1
  2-D Lookup Table4/1 -> [C2_t_ch]
  [SoC_t] -> 1-D Lookup Table/1
  [R0_t_ch] -> Scope5/1
  [SoC_t] -> 2-D Lookup Table/2
  [R0_t_ch] -> Divide5/1
  [I_t] -> Divide7/2
  [C2_t_ch] -> Divide10/1, Divide11/2
  Add3/1 -> Integrator2/1
  [V_t] -> Add11/1
  [Q_t] -> Scope3/1
  [I_t] -> Divide5/2
  [SoC_t] -> 2-D Lookup Table3/2
  1/(Rc*Cs)/1 -> Add3/2
  [OCV_t] -> To Workspace12/1, Scope1/1
  [C1_t_ch] -> Scope13/1
  [Tc_t] -> Scope6/1
  Divide8/1 -> Add9/1
  [OCV_t] -> Add11/2
  [V1_t] -> Divide6/3
  [Ts_t] -> Add4/1
  [Tc_t] -> 2-D Lookup Table1/1
  [C1_t_ch] -> Divide8/2, Divide6/1
  [Tc_t] -> 2-D Lookup Table3/1
  Gain2/1 -> Integrator5/1
  Add8/1 -> 1/(Rc*Cc)/1
  [R1_t_ch] -> Divide6/2
  [R2_t_ch] -> Scope12/1
  [Q_t] -> Cc/1
  Add6/1 -> Integrator3/1
  [R2_t_ch] -> Divide10/2
  [Ts_t] -> Add8/1
  2-D Lookup Table2/1 -> [R2_t_ch]
  Divide11/1 -> Add10/1
  [C2_t_ch] -> Scope14/1
  Add7/1 -> [V_t], To Workspace8/1
  [SoC_t] -> 2-D Lookup Table2/2
  Integrator3/1 -> To Workspace6/1, [Tc_t]
  [Ts_t] -> Add5/2
  [Tc_t] -> Add8/2
  [I_t] -> Divide8/1
  Integrator6/1 -> To Workspace4/1, [V2_t]
  Integrator5/1 -> To Workspace/1, [SoC_t]  "SoC_t"
  Integrator1/1 -> To Workspace3/1, [V1_t]
  [SoC_t] -> Scope2/1
  Constant6/1 -> Add5/1
  2-D Lookup Table1/1 -> [R1_t_ch]
  [SoC_t] -> 2-D Lookup Table4/2
  1/(Ru*Cs)/1 -> Add3/1
  [I_t] -> Gain2/1
  [Tc_t] -> 2-D Lookup Table4/1
  [OCV_t] -> Add7/2
  [V1_t] -> Add7/3
  [I_t] -> Gain1/1
  Integrator4/1 -> To Workspace2/1
  Gain1/1 -> Integrator4/1
  Integrator2/1 -> To Workspace5/1, [Ts_t]
  [I_t] -> Compare To Constant/1
  Compare To Constant/1 -> Stop Simulation/1
  [V1_t] -> MATLAB Function1/3(V1_t)
  [R0_t_ch] -> MATLAB Function1/5(R0_t_ch)
  [OCV_t] -> MATLAB Function1/2(OCV_t)
  [V_t] -> MATLAB Function1/1(V_t)
  [V2_t] -> MATLAB Function1/4(V2_t)
  From26/1 -> Compare To Constant1/1
  Compare To Constant1/1 -> Stop Simulation1/1
  Constant12/1 -> Integrator2/2
  Constant8/1 -> Integrator1/2
  Constant11/1 -> Integrator6/2
  Constant13/1 -> Integrator3/2
  Constant14/1 -> MATLAB Function1/7(C_As)
  Constant15/1 -> MATLAB Function1/8(I_c)
  Constant5/1 -> MATLAB Function1/6(V_max)
  MATLAB Function1/1(I_t) -> To Workspace7/1, [I_t]
  Constant7/1 -> Integrator5/2
  [V_t] -> Scope/1
  [V1_t] -> Scope8/1
  [SoC_t] -> 2-D Lookup Table5/1
  2-D Lookup Table5/1 -> [L0_t_ch]
  Derivative/1 -> Divide/2
  [L0_t_ch] -> Divide/1
  [I_t] -> Derivative/1
  Divide/1 -> Add7/5

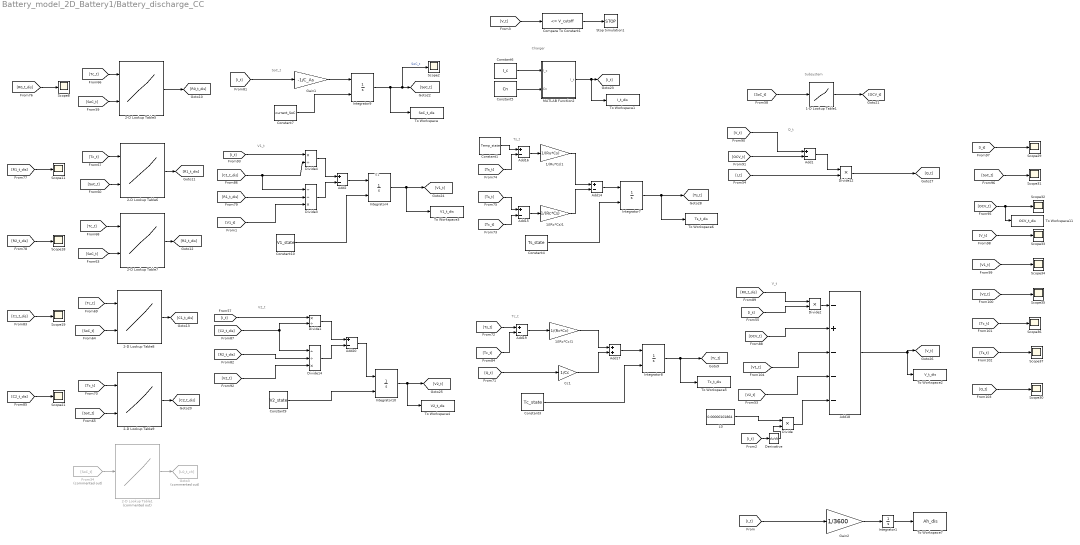
== system Battery_model_2D_Battery1/Battery_discharge_CC ==
  note: Q_t
  note: V1
  note: SoC_t
  note: V1_t
  note: V2_t
  note: V_t
  note: Ts_t
  note: Tc_t
  note: Subsystem
  note: Charger
  1-D Lookup Table1 : Lookup_n-D  NumberOfTableDimensions=1  BreakpointsForDimension1=SoC  BreakpointsForDimension2=Temp  Table=OCV  InternalRulePriority=Speed  RndMeth=Simplest
  1/(Rc*Cc)1 : Gain  Gain=1/(Rc*Cc)
  1/(Rc*Cs)1 : Gain  Gain=1/(Rc*Cs)
  1/(Ru*Cs)1 : Gain  Gain=1/(Ru*Cs)
  2-D Lookup Table1 : Lookup_n-D  Commented=on  NumberOfTableDimensions=1  BreakpointsForDimension1=Temp  BreakpointsForDimension2=SoC  Table=C2_ch  InternalRulePriority=Speed  RndMeth=Simplest
  2-D Lookup Table5 : Lookup_n-D  BreakpointsForDimension1=Temp  BreakpointsForDimension2=SoC  Table=R0_dis  InternalRulePriority=Speed  RndMeth=Simplest
      settings: InputPortMap=u0,u1
  2-D Lookup Table6 : Lookup_n-D  BreakpointsForDimension1=Temp  BreakpointsForDimension2=SoC  Table=R1_dis  InternalRulePriority=Speed  RndMeth=Simplest
      settings: InputPortMap=u0,u1
  2-D Lookup Table7 : Lookup_n-D  BreakpointsForDimension1=Temp  BreakpointsForDimension2=SoC  Table=R2_dis  InternalRulePriority=Speed  RndMeth=Simplest
      settings: InputPortMap=u0,u1
  2-D Lookup Table8 : Lookup_n-D  BreakpointsForDimension1=Temp  BreakpointsForDimension2=SoC  Table=C1_dis  InternalRulePriority=Speed  RndMeth=Simplest
      settings: InputPortMap=u0,u1
  2-D Lookup Table9 : Lookup_n-D  BreakpointsForDimension1=Temp  BreakpointsForDimension2=SoC  Table=C2_dis  InternalRulePriority=Speed  RndMeth=Simplest
      settings: InputPortMap=u0,u1
  Add{1..2,14..16,19..20} (7 alike) : Sum  Inputs=+-
  Add17 : Sum
  Add18 : Sum  Inputs=-+---
  Cc1 : Gain  Gain=1/Cc
  Compare To Constant1 : simulink/Logic and Bit Operations/Compare To Constant  relop=<=  const=V_cutoff  OutDataTypeStr=boolean
  Constant1 : Constant  Value=Temp_state
  Constant10 : Constant  Value=V1_state
  Constant3 : Constant  Value=Tc_state
  Constant4 : Constant  Value=Ts_state
  Constant5 : Constant  Value=Cn
  Constant6 : Constant  Value=I_c
  Constant7 : Constant  Value=current_SoC
  Constant9 : Constant  Value=V2_state
  Derivative : Derivative
  Divide : Product  Inputs=**
  Divide1 : Product  Inputs=*/
  Divide12 : Product  Inputs=**
  Divide14 : Product  Inputs=//*
  Divide2 : Product  Inputs=**
  Divide3 : Product  Inputs=//*
  Divide4 : Product  Inputs=*/
  From34 : From  Commented=on  GotoTag=SoC_t
  Gain1 : Gain  Gain=-1/C_As
  Gain2 : Gain  Gain=1/3600
  Goto3 : Goto  Commented=on  GotoTag=L0_t_ch
  Integrator1 : Integrator
  Integrator{4,7..8,10} (4 alike) : Integrator  InitialConditionSource=external
  Integrator9 : Integrator  InitialConditionSource=external  InitialCondition=V1_ini
  L0 : Constant  Value=0.00000101864
  MATLAB Function2 : MATLAB Function  TreatAsAtomicUnit=on
  Scope{2,8,11,18..19,21,29..37} (15 alike) : Scope
      Scope11 settings: ActiveDisplayYMinimum=-0.125  ActiveDisplayYMaximum=1.125  DataLoggingVariableName=ScopeData7
      Scope18 settings: ActiveDisplayYMinimum=-0.125  ActiveDisplayYMaximum=1.125  DataLoggingVariableName=ScopeData8
      Scope19 settings: ActiveDisplayYMinimum=-0.125  ActiveDisplayYMaximum=1.125  DataLoggingVariableName=ScopeData9
      Scope2 settings: ActiveDisplayYMinimum=-1  ActiveDisplayYMaximum=1
      Scope21 settings: ActiveDisplayYMinimum=-0.125  ActiveDisplayYMaximum=1.125  DataLoggingVariableName=ScopeData10
      Scope29 settings: ActiveDisplayYMinimum=-0.012532  ActiveDisplayYMaximum=0.16806  DataLoggingVariableName=ScopeData15
      Scope30 settings: ActiveDisplayYMinimum=-0.17004  ActiveDisplayYMaximum=1.5304  DataLoggingVariableName=ScopeData23
      Scope31 settings: ActiveDisplayYMinimum=-0.037306  ActiveDisplayYMaximum=0.031954  DataLoggingVariableName=ScopeData16
      Scope32 settings: ActiveDisplayYMinimum=2.8624  ActiveDisplayYMaximum=4.3229  DataLoggingVariableName=ScopeData17
      Scope33 settings: ActiveDisplayYMinimum=2.8623  ActiveDisplayYMaximum=3.1057  DataLoggingVariableName=ScopeData18
      Scope34 settings: ActiveDisplayYMinimum=4.0625E-5  ActiveDisplayYMaximum=0.012439  DataLoggingVariableName=ScopeData19
      Scope35 settings: ActiveDisplayYMinimum=0.00072388  ActiveDisplayYMaximum=0.0085292  DataLoggingVariableName=ScopeData20
      Scope36 settings: ActiveDisplayYMinimum=-4.1824  ActiveDisplayYMaximum=42.6414  DataLoggingVariableName=ScopeData21
      Scope37 settings: ActiveDisplayYMinimum=2.2586  ActiveDisplayYMaximum=3.6824  DataLoggingVariableName=ScopeData22
      Scope8 settings: ActiveDisplayYMinimum=-0.125  ActiveDisplayYMaximum=1.125  DataLoggingVariableName=ScopeData6
  Stop Simulation1 : Stop
  To Workspace : ToWorkspace  VariableName=SoC_t_dis  SampleTime=-1
      settings: Save2DSignal=2-D array (concatenate along first dimension)
  To Workspace1 : ToWorkspace  VariableName=I_t_dis  SaveFormat=Timeseries  SampleTime=-1
  To Workspace11 : ToWorkspace  VariableName=OCV_t_dis  SaveFormat=Timeseries  SampleTime=-1
  To Workspace2 : ToWorkspace  VariableName=V_t_dis  SaveFormat=Timeseries  SampleTime=-1
  To Workspace3 : ToWorkspace  VariableName=V1_t_dis  SampleTime=-1
      settings: Save2DSignal=2-D array (concatenate along first dimension)
  To Workspace4 : ToWorkspace  VariableName=V2_t_dis  SampleTime=-1
      settings: Save2DSignal=2-D array (concatenate along first dimension)
  To Workspace5 : ToWorkspace  VariableName=Tc_t_dis  SampleTime=-1
      settings: Save2DSignal=2-D array (concatenate along first dimension)
  To Workspace6 : ToWorkspace  VariableName=Ts_t_dis  SampleTime=-1
      settings: Save2DSignal=2-D array (concatenate along first dimension)
  To Workspace7 : ToWorkspace  VariableName=Ah_dis  SampleTime=-1
      settings: Save2DSignal=2-D array (concatenate along first dimension)
  wires:
  2-D Lookup Table9/1 -> [C2_t_dis]
  [SoC_t] -> 2-D Lookup Table9/2
  Add18/1 -> [V_t], To Workspace2/1
  [V2_t] -> Scope35/1
  Cc1/1 -> Add17/2
  Divide1/1 -> Add20/1
  1-D Lookup Table1/1 -> [OCV_t]
  [SoC_t] -> Scope31/1
  Gain1/1 -> Integrator9/1
  [Tc_t] -> 2-D Lookup Table5/1
  [OCV_t] -> Add18/2
  Integrator10/1 -> To Workspace4/1, [V2_t]
  1/(Rc*Cc)1/1 -> Add17/1
  [R0_t_dis] -> Scope8/1
  Integrator4/1 -> To Workspace3/1, [V1_t]
  Divide4/1 -> Add2/1
  [Ts_t] -> Add19/1
  [C2_t_dis] -> Divide14/1, Divide1/2
  [V2_t] -> Divide14/3
  1/(Ru*Cs)1/1 -> Add14/1
  [SoC_t] -> 2-D Lookup Table8/2
  Add17/1 -> Integrator8/1
  [Tc_t] -> Scope36/1
  Constant1/1 -> Add16/1
  Divide12/1 -> [Q_t]
  2-D Lookup Table8/1 -> [C1_t_dis]
  Integrator7/1 -> To Workspace6/1, [Ts_t]
  1/(Rc*Cs)1/1 -> Add14/2
  [R1_t_dis] -> Scope11/1
  [Ts_t] -> Add16/2
  [V1_t] -> Add18/3
  Add16/1 -> 1/(Ru*Cs)1/1
  Add1/1 -> Divide12/1
  [I_t] -> Scope29/1
  Divide14/1 -> Add20/2
  [R2_t_dis] -> Divide14/2
  [Q_t] -> Scope30/1
  Add14/1 -> Integrator7/1
  Add2/1 -> Integrator4/1
  [Tc_t] -> 2-D Lookup Table7/1
  [V1_t] -> Scope34/1
  2-D Lookup Table7/1 -> [R2_t_dis]
  2-D Lookup Table6/1 -> [R1_t_dis]
  [V2_t] -> Add18/4
  [SoC_t] -> 2-D Lookup Table6/2
  [R2_t_dis] -> Scope18/1
  [SoC_t] -> 2-D Lookup Table5/2
  2-D Lookup Table5/1 -> [R0_t_dis]
  [OCV_t] -> To Workspace11/1, Scope32/1
  [Q_t] -> Cc1/1
  Divide3/1 -> Add2/2
  [I_t] -> Divide12/2
  Add19/1 -> 1/(Rc*Cc)1/1
  Add20/1 -> Integrator10/1
  [C1_t_dis] -> Scope19/1
  Divide2/1 -> Add18/1
  Add15/1 -> 1/(Rc*Cs)1/1
  [R1_t_dis] -> Divide3/2
  [C1_t_dis] -> Divide4/2, Divide3/1
  Integrator9/1 -> To Workspace/1, Scope2/1, [SoC_t]  "SoC_t"
  [Tc_t] -> Add15/2
  [OCV_t] -> Add1/2
  [C2_t_dis] -> Scope21/1
  [Tc_t] -> 2-D Lookup Table8/1
  [V1_t] -> Divide3/3
  [Tc_t] -> 2-D Lookup Table9/1
  [Ts_t] -> Add15/1
  [Ts_t] -> Scope37/1
  [V_t] -> Scope33/1
  [SoC_t] -> 1-D Lookup Table1/1
  [SoC_t] -> 2-D Lookup Table7/2
  [Tc_t] -> 2-D Lookup Table6/1
  [R0_t_dis] -> Divide2/1
  Integrator8/1 -> To Workspace5/1, [Tc_t]
  [V_t] -> Add1/1
  Constant10/1 -> Integrator4/2
  Constant4/1 -> Integrator7/2
  Constant9/1 -> Integrator10/2
  Constant3/1 -> Integrator8/2
  Integrator1/1 -> To Workspace7/1
  Gain2/1 -> Integrator1/1
  Constant5/1 -> MATLAB Function2/2(Cn)
  Constant6/1 -> MATLAB Function2/1(I_c)
  MATLAB Function2/1(I_t) -> To Workspace1/1, [I_t]
  [V_t] -> Compare To Constant1/1
  Compare To Constant1/1 -> Stop Simulation1/1
  [I_t] -> Gain1/1
  [Tc_t] -> Add19/2
  [I_t] -> Gain2/1
  [I_t] -> Divide4/1
  [I_t] -> Divide1/1
  [I_t] -> Divide2/2
  Constant7/1 -> Integrator9/2
  From34/1 -> 2-D Lookup Table1/1
  2-D Lookup Table1/1 -> Goto3/1
  Derivative/1 -> Divide/2
  Divide/1 -> Add18/5
  [I_t] -> Derivative/1
  L0/1 -> Divide/1
